simulink model "P4"  (R2020b)
settings: Solver=VariableStepAuto  StartTime=0.0  StopTime=10.0  RelTol=1e-3
settings Model: Creator=abdullah  LastModifiedBy=abdullah

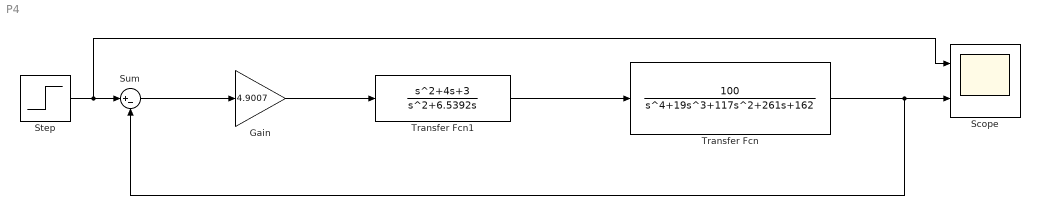
== system P4 ==
  Gain : Gain  Gain=4.9007
  Scope : Scope  NumInputPorts=2
  Step : Step  SampleTime=0
  Sum : Sum  Inputs=|+-
  Transfer Fcn : TransferFcn  Numerator=[100]  Denominator="[ 1    19   117   261   162]"
  Transfer Fcn1 : TransferFcn  Numerator=[1 4 3]  Denominator=[1 6.5392 0]
  wires:
  Transfer Fcn/1 -> Sum/2, Scope/2
  Step/1 -> Scope/1, Sum/1
  Sum/1 -> Gain/1
  Gain/1 -> Transfer Fcn1/1
  Transfer Fcn1/1 -> Transfer Fcn/1
